simulink model "digital"  (R2018a)
settings: Solver=ode4  StartTime=0.0  StopTime=10.0  FixedStep=1e-3  RelTol=1e-3
settings Model: Creator=User  LastModifiedBy=User

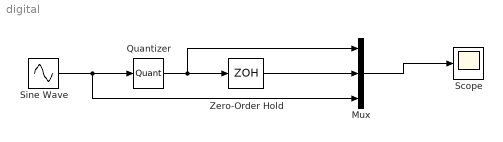
== system digital ==
  Mux : Mux  Inputs=3
  Quantizer : Quantizer
  Scope : Scope
  Sine Wave : Sin  Amplitude=2  SampleTime=0
  Zero-Order Hold : ZeroOrderHold  SampleTime=0.5
  wires:
  Mux/1 -> Scope/1
  Zero-Order Hold/1 -> Mux/2
  Quantizer/1 -> Mux/1, Zero-Order Hold/1
  Sine Wave/1 -> Mux/3, Quantizer/1
